simulink model "optimiser_test_model"  (R2020b)
settings: Solver=VariableStepAuto  StartTime=0.0  StopTime=10.0  RelTol=1e-3
settings Model: Creator=marcus  LastModifiedBy=joeoc
settings SFSimCC: SimCustomHeaderCode="#include \"src/process_optimiser.h\""  SimUserSources=src/process_optimiser.cc  SimAnalyzeCustomCode=on  SimTargetLang=C++

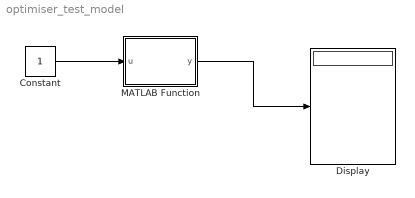
== system optimiser_test_model ==
  Constant : Constant
  Display : Display
  MATLAB Function : MATLAB Function  TreatAsAtomicUnit=on
  wires:
  Constant/1 -> MATLAB Function/1(u)
  MATLAB Function/1(y) -> Display/1

== matlab function optimiser_test_model/MATLAB Function ==
  data: u input; y output double size=3
function y = fcn(u)
    x = [-1; -1; -1];
    z = false;
    
    box_points = [0 0 0 1 2 3];
    item_points = [4 2 1 1 2 4 1 0 0 4 4 4];
    item_indices = [0 6];
    dimensions = [10 10 10];
    
    z = coder.ceval("process_optimiser_main", box_points, item_points, size(item_points, 2), item_indices, size(item_indices, 2), dimensions, coder.wref(x))
    
y = x;
